simulink model "DT_SigmaDelta"  (Simulink 7.9)
settings: Solver=VariableStepDiscrete  StartTime=0.0  StopTime=1  RelTol=1e-6
PreLoadFcn:
  | load one_stage.mat
undefined symbols (not defined in the file or in its folder): DiscIntNeverNeededParam
libraries: dspmlti4 x21, simulink x3, dspvision x1
(part 6 of 13)

== system DT_SigmaDelta/Decimation4 ==
  Bit Stream In : Inport
  Bit Stream In1 : Inport  Port=2
  One Stage Decimation Digital Filter : dspmlti4/FIR Decimation  Tag=BlockMethodSubSystem  RequirementInfo={'other' 'AD1877.pdf' '#4' 'true' 'ADI AD1877 Data Sheet' '' } %GIDa_c24f116f_3404_4c47_89cb_6d2a7f856a4b  h=[1.55406407911568e-005 -4.02976869344532e-006 -3.62744882919974e-006 -3.32415900794419e-006 -3.10004007346292e-006 -2.94488775900927e-006 -2.84407867825443e-006 -2.79175810569639e-006 -2.77680534274625e-006 -2.79636876946116e-006 -2.84159739559419e-006 -2.91172216432913e-006 -2.99938731666961e-006 -3.10526988821609e-006 -3.22293122491583e-006 -3.35411175577608e-006 -3.49288760841827e-006 -3.64182441067023e-006 -3.79519422790614e-006 -3.95625120366779e-006 -4.11924776887857e-006 -4.28807690784027e-006 -4.45674935295447e-006 -4.62985561457222e-006 -4.800897058436e-006 -4.9753188968358e-006 -5.14579209170125e-006 -5.31896147362731e-006 -5.48613787011061e-006 -5.65584148286576e-006 -5.81687994870294e-006 -5.98156442936665e-006 -6.1319779994032e-006 -6.29670705116336e-006 -6.41916030653874e-006 -6.5873274394144e-006 -6.7177176233061e-006 -6.82652503989139e-006 -6.95495460798152e-006 -7.07534295461106e-006 -7.1850354195168e-006 -7.27502374181979e-006 -7.35666591949478e-006 -7.42908966098812e-006 -7.49731879243244e-006 -7.55554016300166e-006 -7.60384694343128e-006 -7.63736428406282e-006 -7.65751209128601e-006 -7.66271823557677e-006 -7.65541155261304e-006 -7.63501627507501e-006 -7.60282107295533e-006 -7.55771586095076e-006 -7.49955110139743e-006 -7.42707797821989e-006 -7.33956971085392e-006 -7.23653893398005e-006 -7.11727392514411e-006 -6.98238367840012e-006 -6.83104946879514e-006 -6.66483440906746e-006 -6.48225897487408e-006 -6.28578538645417e-006 -6.07254142810829e-006 -5.84668058135014e-006 -5.60212405026277e-006 -5.34827643472346e-006 -5.07102301413336e-006 -4.78659690402004e-006 -4.48580556034723e-006 -4.16155600384522e-006 -3.83401955134294e-006 -3.48874328670483e-006 -3.12800075717904e-006 -2.75159431264472e-006 -2.36710798789534e-006 -1.97052071697094e-006 -1.56289826517329e-006 -1.1415501968765e-006 -7.10846494538715e-007 -2.70732289220279e-007 1.75793679903884e-007 6.30605543525479e-007 1.09226506478532e-006 1.56189731593155e-006 2.03697170915753e-006 2.51723717113145e-006 3.00015723143587e-006 3.48579071809432e-006 3.9725933377886e-006 4.46080384428176e-006 4.9490441253173e-006 5.43679761975195e-006 5.92239585030302e-006 6.40461366377309e-006 6.88208470617973e-006 7.35331974962638e-006 7.81788083672163e-006 8.27366149467831e-006 8.72161880365281e-006 9.15789014754869e-006 9.58466277051695e-006 9.99868488513386e-006 1.03961241773662e-005 1.07845165019174e-005 1.11507237228684e-005 1.1501595755956e-005 1.18347779752421e-005 1.21491508417921e-005 1.24402661260835e-005 1.27113476734474e-005 1.29603423782727e-005 1.31870907689413e-005 1.33876586413025e-005 1.35630197026232e-005 1.37115784405412e-005 1.38343308497875e-005 1.39285220410779e-005 1.39941223446797e-005 1.40289966823036e-005 1.40342134443906e-005 1.40084936488381e-005 1.39526353305602e-005 1.3864821369379e-005 1.37453066068296e-005 1.35925703287186e-005 1.34073463479953e-005 1.3188789625357e-005 1.29377174450497e-005 1.26533131128865e-005 1.23359924862388e-005 1.19851377636711e-005 1.16010858578809e-005 1.11839953027825e-005 1.07344849783013e-005 1.02524591509204e-005 9.74071213530745e-006 9.19501972815777e-006 8.62303106439748e-006 8.0182133965873e-006 7.38519650181956e-006 6.72464037253548e-006 6.03717286198122e-006 5.32193639834688e-006 4.58308951056204e-006 3.82060966862603e-006 3.03594631004846e-006 2.22877471347222e-006 1.40249577164911e-006 5.57771396078279e-007 -3.03081212010611e-007 -1.18011136255105e-006 -2.0703284116168e-006 -2.97257001796215e-006 -3.8836096780257e-006 -4.80290798314314e-006 -5.72785477296596e-006 -6.65770229898759e-006 -7.58923677050474e-006 -8.52121235074221e-006 -9.45049303838782e-006 -1.03761550722017e-005 -1.12952557815384e-005 -1.22066400703126e-005 -1.31069929510391e-005 -1.39948646063552e-005 -1.48669844016962e-005 -1.5722291797911e-005 -1.6557361960285e-005 -1.73721743499725e-005 -1.81614198379814e-005 -1.89271227804299e-005 -1.96621709077627e-005 -2.03681220570147e-005 -2.10414746689456e-005 -2.16795973059757e-005 ...(+43466 chars)]  D=64  filtStruct=Direct form  framing=Maintain input frame size  inputOffset=0  outputBufInitCond=0  InputProcessing=Inherited (this choice will be removed - see release notes)  firstCoeffDataTypeStr=Inherit: Same word length as input  firstCoeffLastDataTypeStr=Inherit: Same word length as input  firstCoeffMin=[]  firstCoeffMax=[]  outputDataTypeStr=Inherit: Same as accumulator  outputLastDataTypeStr=Inherit: Same as accumulator  outputMin=[]  outputMax=[]  roundingMode=Floor  overflowMode=off  FilterSource=Filter object  FilterObject=h
  One Stage Decimation Digital Filter1 : dspmlti4/FIR Decimation  Tag=BlockMethodSubSystem  RequirementInfo={'other' 'AD1877.pdf' '#4' 'true' 'ADI AD1877 Data Sheet' '' } %GIDa_3c4c1e4f_4e0d_443a_adae_fc9c11491011  h=[1.55406407911568e-005 -4.02976869344532e-006 -3.62744882919974e-006 -3.32415900794419e-006 -3.10004007346292e-006 -2.94488775900927e-006 -2.84407867825443e-006 -2.79175810569639e-006 -2.77680534274625e-006 -2.79636876946116e-006 -2.84159739559419e-006 -2.91172216432913e-006 -2.99938731666961e-006 -3.10526988821609e-006 -3.22293122491583e-006 -3.35411175577608e-006 -3.49288760841827e-006 -3.64182441067023e-006 -3.79519422790614e-006 -3.95625120366779e-006 -4.11924776887857e-006 -4.28807690784027e-006 -4.45674935295447e-006 -4.62985561457222e-006 -4.800897058436e-006 -4.9753188968358e-006 -5.14579209170125e-006 -5.31896147362731e-006 -5.48613787011061e-006 -5.65584148286576e-006 -5.81687994870294e-006 -5.98156442936665e-006 -6.1319779994032e-006 -6.29670705116336e-006 -6.41916030653874e-006 -6.5873274394144e-006 -6.7177176233061e-006 -6.82652503989139e-006 -6.95495460798152e-006 -7.07534295461106e-006 -7.1850354195168e-006 -7.27502374181979e-006 -7.35666591949478e-006 -7.42908966098812e-006 -7.49731879243244e-006 -7.55554016300166e-006 -7.60384694343128e-006 -7.63736428406282e-006 -7.65751209128601e-006 -7.66271823557677e-006 -7.65541155261304e-006 -7.63501627507501e-006 -7.60282107295533e-006 -7.55771586095076e-006 -7.49955110139743e-006 -7.42707797821989e-006 -7.33956971085392e-006 -7.23653893398005e-006 -7.11727392514411e-006 -6.98238367840012e-006 -6.83104946879514e-006 -6.66483440906746e-006 -6.48225897487408e-006 -6.28578538645417e-006 -6.07254142810829e-006 -5.84668058135014e-006 -5.60212405026277e-006 -5.34827643472346e-006 -5.07102301413336e-006 -4.78659690402004e-006 -4.48580556034723e-006 -4.16155600384522e-006 -3.83401955134294e-006 -3.48874328670483e-006 -3.12800075717904e-006 -2.75159431264472e-006 -2.36710798789534e-006 -1.97052071697094e-006 -1.56289826517329e-006 -1.1415501968765e-006 -7.10846494538715e-007 -2.70732289220279e-007 1.75793679903884e-007 6.30605543525479e-007 1.09226506478532e-006 1.56189731593155e-006 2.03697170915753e-006 2.51723717113145e-006 3.00015723143587e-006 3.48579071809432e-006 3.9725933377886e-006 4.46080384428176e-006 4.9490441253173e-006 5.43679761975195e-006 5.92239585030302e-006 6.40461366377309e-006 6.88208470617973e-006 7.35331974962638e-006 7.81788083672163e-006 8.27366149467831e-006 8.72161880365281e-006 9.15789014754869e-006 9.58466277051695e-006 9.99868488513386e-006 1.03961241773662e-005 1.07845165019174e-005 1.11507237228684e-005 1.1501595755956e-005 1.18347779752421e-005 1.21491508417921e-005 1.24402661260835e-005 1.27113476734474e-005 1.29603423782727e-005 1.31870907689413e-005 1.33876586413025e-005 1.35630197026232e-005 1.37115784405412e-005 1.38343308497875e-005 1.39285220410779e-005 1.39941223446797e-005 1.40289966823036e-005 1.40342134443906e-005 1.40084936488381e-005 1.39526353305602e-005 1.3864821369379e-005 1.37453066068296e-005 1.35925703287186e-005 1.34073463479953e-005 1.3188789625357e-005 1.29377174450497e-005 1.26533131128865e-005 1.23359924862388e-005 1.19851377636711e-005 1.16010858578809e-005 1.11839953027825e-005 1.07344849783013e-005 1.02524591509204e-005 9.74071213530745e-006 9.19501972815777e-006 8.62303106439748e-006 8.0182133965873e-006 7.38519650181956e-006 6.72464037253548e-006 6.03717286198122e-006 5.32193639834688e-006 4.58308951056204e-006 3.82060966862603e-006 3.03594631004846e-006 2.22877471347222e-006 1.40249577164911e-006 5.57771396078279e-007 -3.03081212010611e-007 -1.18011136255105e-006 -2.0703284116168e-006 -2.97257001796215e-006 -3.8836096780257e-006 -4.80290798314314e-006 -5.72785477296596e-006 -6.65770229898759e-006 -7.58923677050474e-006 -8.52121235074221e-006 -9.45049303838782e-006 -1.03761550722017e-005 -1.12952557815384e-005 -1.22066400703126e-005 -1.31069929510391e-005 -1.39948646063552e-005 -1.48669844016962e-005 -1.5722291797911e-005 -1.6557361960285e-005 -1.73721743499725e-005 -1.81614198379814e-005 -1.89271227804299e-005 -1.96621709077627e-005 -2.03681220570147e-005 -2.10414746689456e-005 -2.16795973059757e-005 ...(+43466 chars)]  D=64  filtStruct=Direct form  framing=Maintain input frame size  inputOffset=0  outputBufInitCond=0  InputProcessing=Inherited (this choice will be removed - see release notes)  firstCoeffDataTypeStr=Inherit: Same word length as input  firstCoeffLastDataTypeStr=Inherit: Same word length as input  firstCoeffMin=[]  firstCoeffMax=[]  outputDataTypeStr=Inherit: Same as accumulator  outputLastDataTypeStr=Inherit: Same as accumulator  outputMin=[]  outputMax=[]  roundingMode=Floor  overflowMode=off  FilterSource=Filter object  FilterObject=h
  Digital Out : Outport
  Digital Out1 : Outport  Port=2
  wires:
  One Stage Decimation Digital Filter1/1 -> Digital Out1/1  "Digital Output 48 KHz"
  Bit Stream In1/1 -> One Stage Decimation Digital Filter1/1
  One Stage Decimation Digital Filter/1 -> Digital Out/1  "Digital Output 48 KHz"
  Bit Stream In/1 -> One Stage Decimation Digital Filter/1
